simulink model "Oppgave3d"  (R2023a)
settings: Solver=VariableStepAuto  StartTime=0.0  StopTime=10.0  RelTol=1e-3
settings Model: Creator=augus  LastModifiedBy=augus

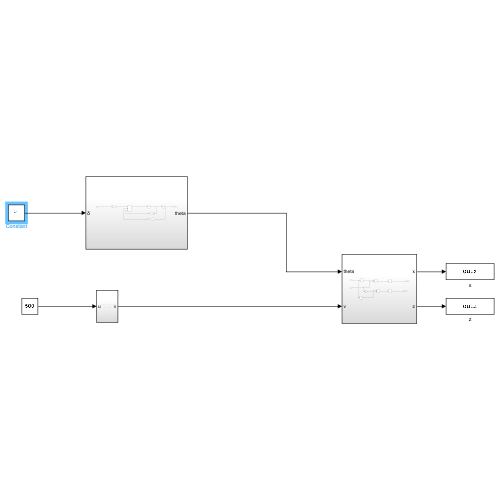
[thumbnail: Simulink's stored preview of the top-level diagram]
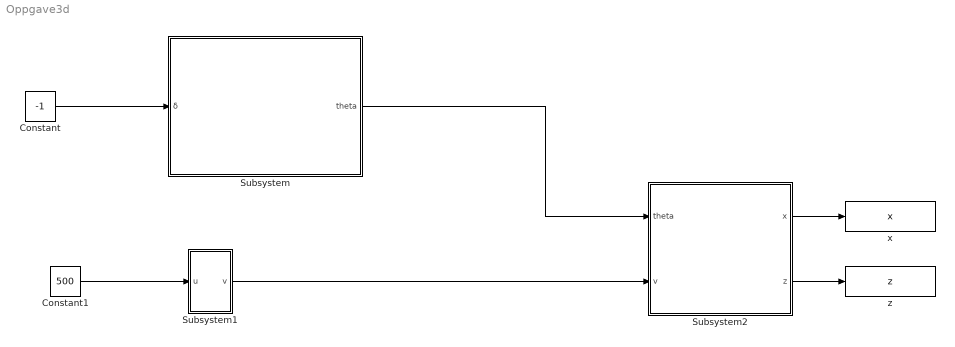
== system Oppgave3d ==
  Constant : Constant  Value=-1
  Constant1 : Constant  Value=500
  Subsystem : Subsystem
  Subsystem1 : Subsystem
  Subsystem2 : Subsystem
  x : ToWorkspace  VariableName=x  SaveFormat=Timeseries  SampleTime=-1
  z : ToWorkspace  VariableName=z  SaveFormat=Timeseries  SampleTime=-1
  wires:
  Subsystem2/2(z) -> z/1
  Constant/1 -> Subsystem/1(δ)
  Constant1/1 -> Subsystem1/1(u)
  Subsystem2/1(x) -> x/1
  Subsystem1/1(v) -> Subsystem2/2(v)
  Subsystem/1(theta) -> Subsystem2/1(theta)

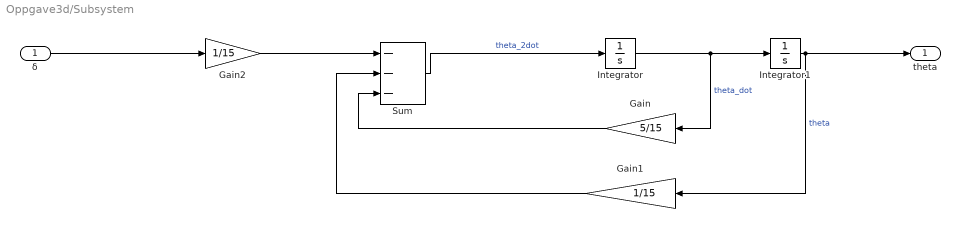
== system Oppgave3d/Subsystem ==
  δ : Inport
  Gain : Gain  Gain=5/15
  Gain1 : Gain  Gain=1/15
  Gain2 : Gain  Gain=1/15
  Integrator : Integrator
  Integrator1 : Integrator
  Sum : Sum  Inputs=---
  theta : Outport
  wires:
  Integrator1/1 -> Gain1/1, theta/1  "theta"
  Integrator/1 -> Gain/1, Integrator1/1  "theta_dot"
  Sum/1 -> Integrator/1  "theta_2dot"
  δ/1 -> Gain2/1
  Gain2/1 -> Sum/1
  Gain/1 -> Sum/3
  Gain1/1 -> Sum/2

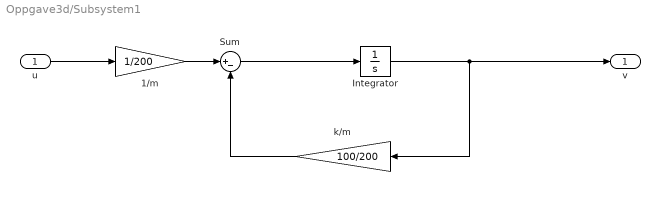
== system Oppgave3d/Subsystem1 ==
  u : Inport
  1/m : Gain  Gain=1/200
  Integrator : Integrator
  Sum : Sum  Inputs=|+-
  k/m : Gain  Gain=100/200
  v : Outport
  wires:
  k/m/1 -> Sum/2
  Integrator/1 -> v/1, k/m/1
  Sum/1 -> Integrator/1
  1/m/1 -> Sum/1
  u/1 -> 1/m/1

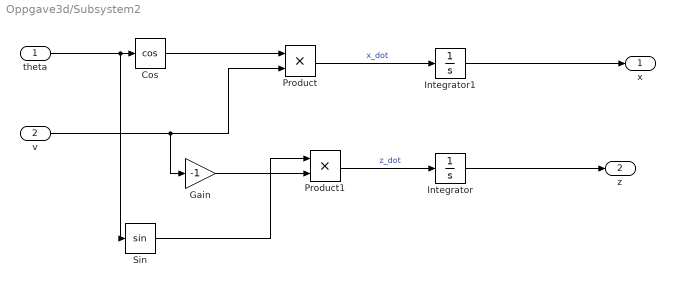
== system Oppgave3d/Subsystem2 ==
  theta : Inport
  v : Inport  Port=2
  Cos : Trigonometry  Operator=cos
  Gain : Gain  Gain=-1
  Integrator : Integrator
  Integrator1 : Integrator
  Product : Product
  Product1 : Product
  Sin : Trigonometry
  x : Outport
  z : Outport  Port=2
  wires:
  theta/1 -> Sin/1, Cos/1
  v/1 -> Gain/1, Product/2
  Cos/1 -> Product/1
  Sin/1 -> Product1/1
  Gain/1 -> Product1/2
  Product1/1 -> Integrator/1  "z_dot"
  Product/1 -> Integrator1/1  "x_dot"
  Integrator/1 -> z/1
  Integrator1/1 -> x/1
